simulink model "pendule_inv_etu"  (R2021a)
settings: Solver=VariableStepAuto  StartTime=0.0  StopTime=10.0  RelTol=1e-3
values from neighbouring files (symbols this model uses):
  K = [10 1]    [simu_pendule_inv_capteur_etu.m]    (also in simu_pendule_inv_echant_etu.m = [30 10]; simu_pendule_inv_etu.m = [30 10])
  ue = 0    [simu_pendule_inv_capteur_etu.m]    (also in simu_pendule_inv_echant_etu.m; simu_pendule_inv_etu.m)
  x0 = [pi/20 0]'    [simu_pendule_inv_capteur_etu.m]    (also in simu_pendule_inv_echant_etu.m; simu_pendule_inv_etu.m = [pi/10 0]')
  xe = [0 0]'    [simu_pendule_inv_capteur_etu.m]    (also in simu_pendule_inv_echant_etu.m; simu_pendule_inv_etu.m)
settings Model: Creator=abennagh  LastModifiedBy=abennagh

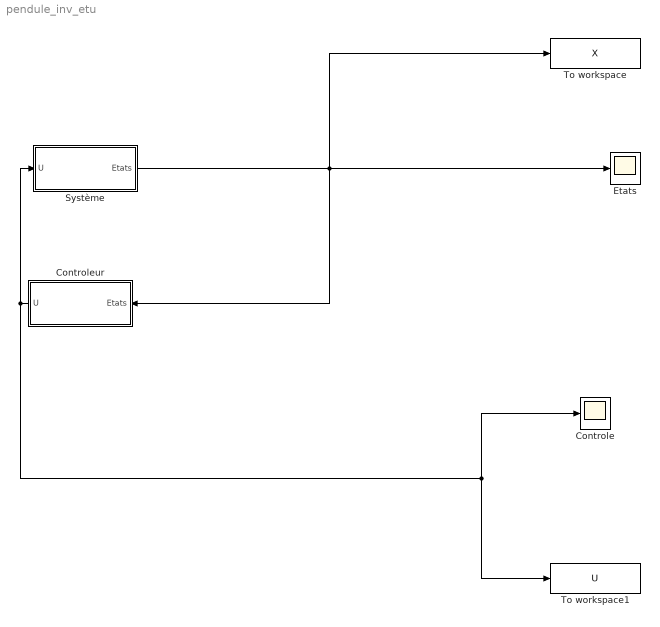
== system pendule_inv_etu ==
  Controle : Scope
  Controleur : Subsystem
  Etats : Scope
  Système : Subsystem
  To workspace : ToWorkspace  VariableName=X  SaveFormat=Timeseries  SampleTime=-1
  To workspace1 : ToWorkspace  VariableName=U  SaveFormat=Timeseries  SampleTime=-1
  wires:
  Controleur/1(U) -> Controle/1, To workspace1/1, Système/1(U)
  Système/1(Etats) -> Controleur/1(Etats), To workspace/1, Etats/1

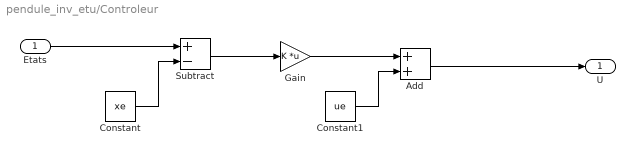
== system pendule_inv_etu/Controleur ==
  Etats : Inport
  Add : Sum
  Constant : Constant  Value=xe  OutDataTypeStr=double
  Constant1 : Constant  Value=ue
  Gain : Gain  Gain=K  Multiplication=Matrix(K*u)
  Subtract : Sum  Inputs=+-
  U : Outport
  wires:
  Constant/1 -> Subtract/2
  Constant1/1 -> Add/2
  Etats/1 -> Subtract/1
  Add/1 -> U/1
  Gain/1 -> Add/1
  Subtract/1 -> Gain/1

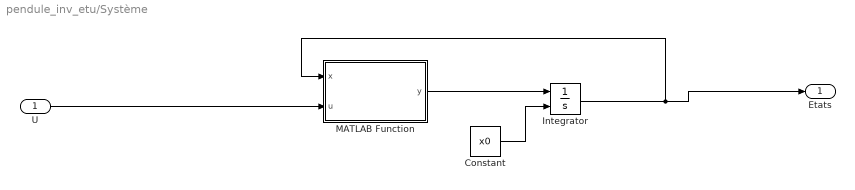
== system pendule_inv_etu/Système ==
  U : Inport
  Constant : Constant  Value=x0
  Integrator : Integrator  InitialConditionSource=external
  MATLAB Function : MATLAB Function  TreatAsAtomicUnit=on
  Etats : Outport
  wires:
  U/1 -> MATLAB Function/2(u)
  Constant/1 -> Integrator/2
  MATLAB Function/1(y) -> Integrator/1
  Integrator/1 -> MATLAB Function/1(x), Etats/1

== matlab function pendule_inv_etu/Système/MATLAB Function ==
  data: x input; u input; y output
function y = fcn(x,u)
g = 9.81; l = 10;   % constantes
y = [x(2); (g/l)*sin(x(1))-(cos(x(1))*u)/l];
